simulink model "feixianxing"  (R2015a)
settings: Solver=ode45  StartTime=0.0  StopTime=0.00002  RelTol=1e-3
libraries: dspquant2 x2, simulink x1
settings Model: Creator=Administrator  LastModifiedBy=Administrator

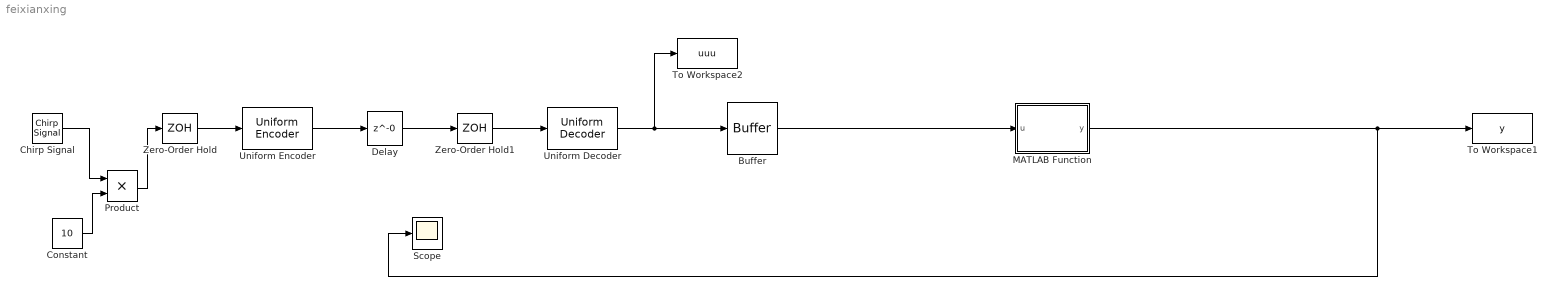
== system feixianxing ==
  Buffer : Buffer  N=2  V=1  TreatMby1Signals=One channel
  Chirp Signal : simulink/Sources/Chirp Signal  f1=1  T=20e-6  f2=10e6
  Constant : Constant  Value=10
  Delay : Delay  DelayLength=0  InitialCondition=0
  MATLAB Function : MATLAB Function  TreatAsAtomicUnit=on
  Product : Product
  Scope : Scope
      settings: TimeRange=2e-05
  To Workspace1 : ToWorkspace  VariableName=y  SampleTime=-1
  To Workspace2 : ToWorkspace  VariableName=uuu  SampleTime=-1
  Uniform Decoder : dspquant2/Uniform Decoder  peak=1  bits=8  overflowMode=Saturate  otype=Double
  Uniform Encoder : dspquant2/Uniform Encoder  peak=1  bits=8  otype=Signed integer
  Zero-Order Hold : ZeroOrderHold  SampleTime=1/50000000
  Zero-Order Hold1 : ZeroOrderHold  SampleTime=1/50000000
  wires:
  Zero-Order Hold/1 -> Uniform Encoder/1
  Uniform Encoder/1 -> Delay/1
  Zero-Order Hold1/1 -> Uniform Decoder/1
  Delay/1 -> Zero-Order Hold1/1
  Buffer/1 -> MATLAB Function/1(u)
  Chirp Signal/1 -> Product/1
  Constant/1 -> Product/2
  Product/1 -> Zero-Order Hold/1
  Uniform Decoder/1 -> Buffer/1, To Workspace2/1
  MATLAB Function/1(y) -> Scope/1, To Workspace1/1

== matlab function feixianxing/MATLAB Function ==
  data: u input; y output
function y = fcn(u)
%#codegen

k=2;%次数
m=1;%阶数
b=[1 0.1;
     0.1 0.1];
 uu=u';


 z=zeros(length(uu),1);

for kk=m+1:length(uu)
 for ii=0:m
    sum=0;
    for jj=1:k
     sum=sum+b(ii+1,jj)*abs(uu(kk-ii)^(2*jj-2))*uu(kk-ii);
    end
    z(kk)=z(kk)+sum;
 end
end
y=z;
return ;
y=z(m+1:length(uu));
